simulink subsystem "Calculate_sumsquares"  (R2023b)
settings: Solver=VariableStepAuto  StartTime=0.0  StopTime=10.0  RelTol=1e-3
undefined symbols (not defined in the file): shuntNumHarmonics
settings Model: Creator=Veimar  LastModifiedBy=Veimar

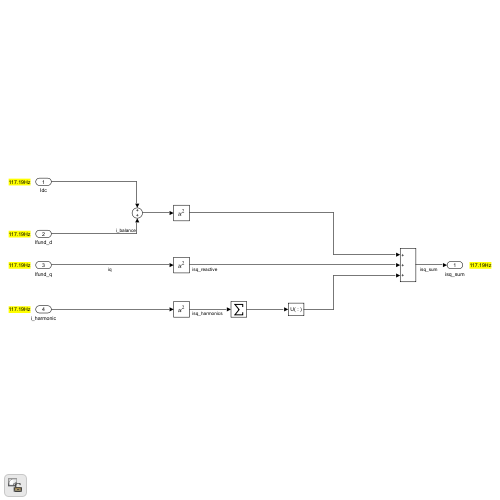
[thumbnail: Simulink's stored preview of the top-level diagram]
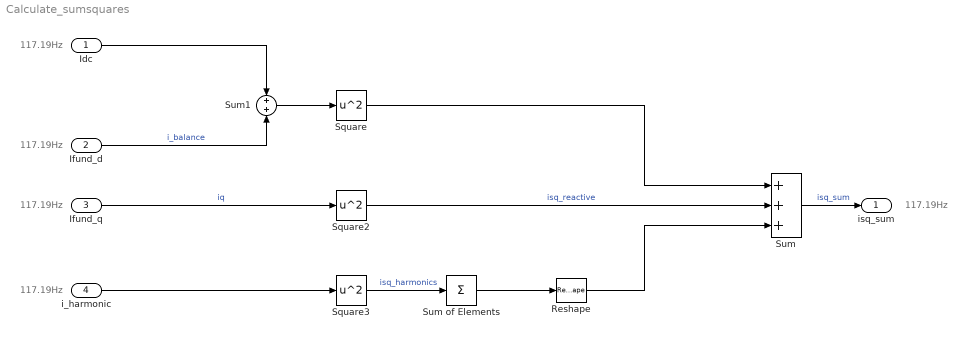
== system Calculate_sumsquares ==
  note: 117.19Hz
  note: 117.19Hz
  note: 117.19Hz
  note: 117.19Hz
  note: 117.19Hz
  Idc : Inport  OutDataTypeStr=single  PortDimensions=3
  Ifund_d : Inport  Port=2  OutDataTypeStr=single  PortDimensions=3
  Ifund_q : Inport  Port=3  OutDataTypeStr=single  PortDimensions=3
  i_harmonic : Inport  Port=4  OutDataTypeStr=single  PortDimensions=[3 shuntNumHarmonics]
  Reshape : Reshape
  Square : Math  Operator=square
  Square2 : Math  Operator=square
  Square3 : Math  Operator=square
  Sum : Sum  Inputs=+++
  Sum of Elements : Sum  Inputs=+  CollapseMode=Specified dimension  CollapseDim=2
  Sum1 : Sum  Inputs=+|+
  isq_sum : Outport  OutDataTypeStr=single  PortDimensions=3
  wires:
  Ifund_d/1 -> Sum1/2  "i_balance"
  Idc/1 -> Sum1/1
  Ifund_q/1 -> Square2/1  "iq"
  Sum1/1 -> Square/1
  Square/1 -> Sum/1
  Square2/1 -> Sum/2  "isq_reactive"
  Sum/1 -> isq_sum/1  "isq_sum"
  i_harmonic/1 -> Square3/1
  Sum of Elements/1 -> Reshape/1
  Reshape/1 -> Sum/3
  Square3/1 -> Sum of Elements/1  "isq_harmonics"
